simulink subsystem "TOAD_StateEstimator_2"  (R2026a)
settings: Solver=VariableStepAuto
undefined symbols (not defined in the file): constants6DoF, dt_SIM
settings Model: Creator=pplat  LastModifiedBy=alex2

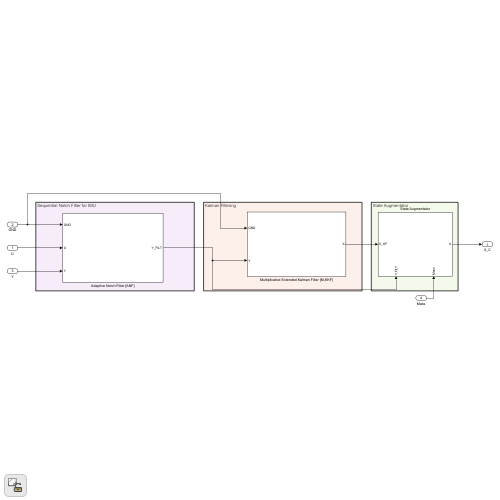
[thumbnail: Simulink's stored preview of the top-level diagram]
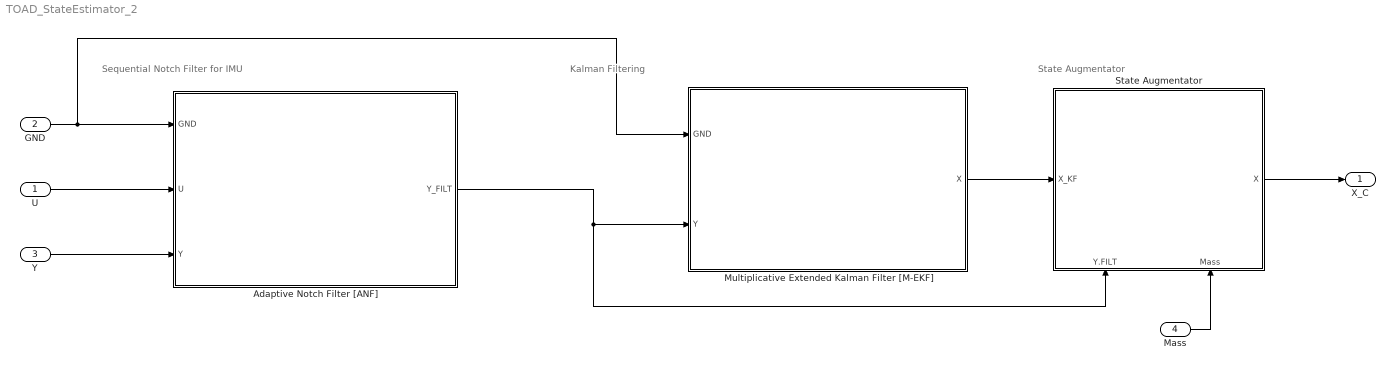
== system TOAD_StateEstimator_2 ==
  note: Kalman Filtering
  note: State Augmentator
  note: Sequential Notch Filter for IMU
  U : Inport  PortDimensions=[4, 1]
  GND : Inport  Port=2
  Y : Inport  Port=3  PortDimensions=[15, 1]
  Mass : Inport  Port=4
  Adaptive Notch Filter [ANF] : Subsystem
  Multiplicative Extended Kalman Filter [M-EKF] : Subsystem
  State Augmentator : Subsystem
      settings: PortSchema="{\"entries\":[{\"content\":{\"sides\":[{\"content\":{\"connectorIds\":[\"In1\"]},\"type\":\"ConnectorPlacement.EquallySpacedRectSide\",\"uuid\":\"bb6458aa-622a-4d42-b468-f616d6e302fe\"},{\"content\":{\"connectorIds\":[\"Out1\"],\"side\":\"RIGHT\"},\"type\":\"ConnectorPlacement.EquallySpacedRectSide\",\"uuid\":\"af8bade2-eb0a-4714-9db5-d33244eb3558\"},{\"content\":{\"side\":\"TOP\"},\"type\":\"ConnectorPlacement.EquallySpacedRectSide\",\"uuid\":\"05a7f106-e447-475e-b3b5-727cb0579a7b\"},{\"content\":{\"connectorIds\":[\"In2\",\"In3\"],\"side\":\"BOTTOM\"},\"type\":\"ConnectorPlacement.EquallySpacedRectSide\",\"uuid\":\"a6d44455-a42d-44f7-b37b-0d3db398c8f2\"}]},\"type\":\"ConnectorPlacement.EquallySpacedConnector\",\"uuid\":\"c6f62579-6b17-43b5-92f1-6190f0d9fd8b\"}],\"packageUris\":[\"http://schema.mathworks.com/mf0/Connector/R2020b\"],\"version\":\"1.0\"}"
  X_C : Outport
  wires:
  Adaptive Notch Filter [ANF]/1(Y_FILT) -> Multiplicative Extended Kalman Filter [M-EKF]/2(Y), State Augmentator/2(Y.FILT)
  Y/1 -> Adaptive Notch Filter [ANF]/3(Y)
  Multiplicative Extended Kalman Filter [M-EKF]/1(X) -> State Augmentator/1(X_KF)
  State Augmentator/1(X) -> X_C/1
  U/1 -> Adaptive Notch Filter [ANF]/2(U)
  GND/1 -> Multiplicative Extended Kalman Filter [M-EKF]/1(GND), Adaptive Notch Filter [ANF]/1(GND)
  Mass/1 -> State Augmentator/3(Mass)

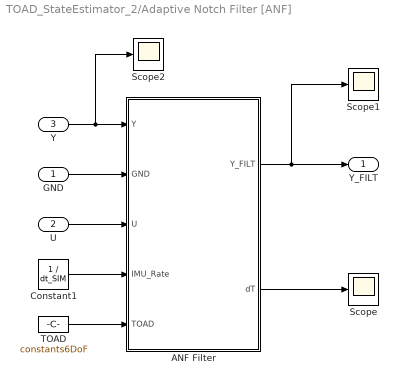
== system TOAD_StateEstimator_2/Adaptive Notch Filter [ANF] ==
  GND : Inport
  U : Inport  Port=2
  Y : Inport  Port=3
  ANF Filter : MATLAB Function  TreatAsAtomicUnit=on
  Constant1 : Constant  Value=1 / dt_SIM
  Scope : Scope
      settings: ActiveDisplayYMinimum=0.00014823443072048078  ActiveDisplayYMaximum=0.0020512828730928742  DataLoggingVariableName=ScopeData12
  Scope1 : Scope
      settings: ActiveDisplayYMinimum=-0.5661858721930958  ActiveDisplayYMaximum=0.35291049526280732  DataLoggingVariableName=ScopeData15
  Scope2 : Scope
      settings: ActiveDisplayYMinimum=-0.41652600912689441  ActiveDisplayYMaximum=0.41641236525722142  DataLoggingVariableName=ScopeData16
  TOAD : Constant  Value=constants6DoF  OutDataTypeStr=Bus: Vehicle_Bus
  Y_FILT : Outport
  wires:
  TOAD/1 -> ANF Filter/5(TOAD)
  ANF Filter/2(dT) -> Scope/1
  Constant1/1 -> ANF Filter/4(IMU_Rate)
  Y/1 -> ANF Filter/1(Y), Scope2/1
  U/1 -> ANF Filter/3(U)
  GND/1 -> ANF Filter/2(GND)
  ANF Filter/1(Y_FILT) -> Y_FILT/1, Scope1/1

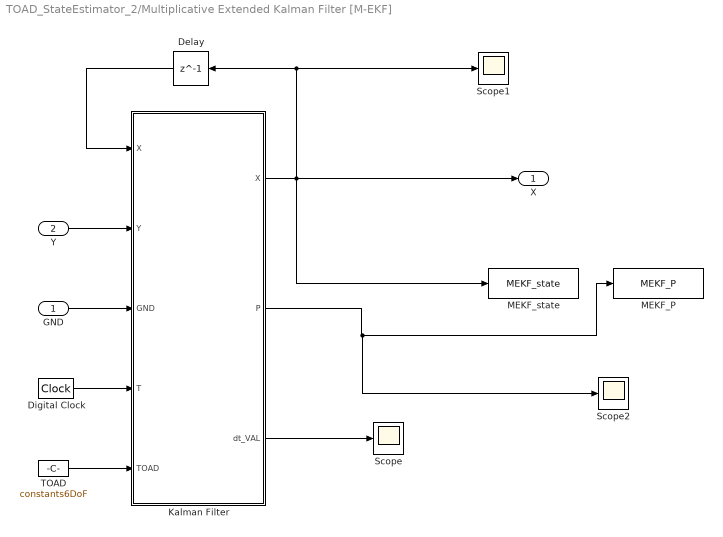
== system TOAD_StateEstimator_2/Multiplicative Extended Kalman Filter [M-EKF] ==
  GND : Inport
  Y : Inport  Port=2
  Delay : Delay  DelayLength=1  InitialCondition=[1; zeros(18,1)]
  Digital Clock : DigitalClock  SampleTime=dt_SIM
  Kalman Filter : MATLAB Function  TreatAsAtomicUnit=on
  MEKF_P : ToWorkspace  VariableName=MEKF_P  SaveFormat=Timeseries  SampleTime=-1
  MEKF_state : ToWorkspace  VariableName=MEKF_state  SaveFormat=Timeseries  SampleTime=-1
  Scope : Scope
      settings: ActiveDisplayYMinimum=-1  ActiveDisplayYMaximum=1
  Scope1 : Scope
      settings: ActiveDisplayYMinimum=-0.012655321840747358  ActiveDisplayYMaximum=0.022187884055420493  DataLoggingVariableName=ScopeData11
  Scope2 : Scope
      settings: ActiveDisplayYMinimum=-0.00099337090493864869  ActiveDisplayYMaximum=0.010796249758337241
  TOAD : Constant  Value=constants6DoF  OutDataTypeStr=Bus: Vehicle_Bus
  X : Outport
  wires:
  Kalman Filter/2(P) -> MEKF_P/1, Scope2/1
  GND/1 -> Kalman Filter/3(GND)
  TOAD/1 -> Kalman Filter/5(TOAD)
  Delay/1 -> Kalman Filter/1("X ")
  Y/1 -> Kalman Filter/2(Y)
  Kalman Filter/1(X) -> MEKF_state/1, X/1, Delay/1, Scope1/1
  Digital Clock/1 -> Kalman Filter/4(T)
  Kalman Filter/3(dt_VAL) -> Scope/1

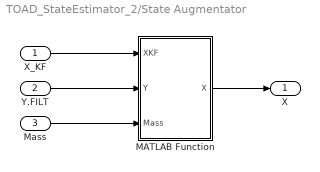
== system TOAD_StateEstimator_2/State Augmentator ==
  X_KF : Inport
  Y.FILT : Inport  Port=2
  Mass : Inport  Port=3
  MATLAB Function : MATLAB Function  TreatAsAtomicUnit=on
  X : Outport
  wires:
  Mass/1 -> MATLAB Function/3(Mass)
  Y.FILT/1 -> MATLAB Function/2(Y)
  MATLAB Function/1(X) -> X/1
  X_KF/1 -> MATLAB Function/1(XKF)

== matlab function TOAD_StateEstimator_2/Multiplicative Extended Kalman Filter [M-EKF]/Kalman Filter ==
  data: X input; Y input; GND input; X output; T input; TOAD input; P output; dt_VAL output
function [X, P, dt_VAL] = MEKF(X, Y, GND, T, TOAD)

    % Measure simulation timestep
    persistent dt lastT lastP
    if isempty(dt)
        dt = 0;
        lastT = 0;
        lastP = eye(18);
    end
    dt = T - lastT;
    lastT = T;
    
    if GND
        [X, lastP] = GroundEstimator(X, TOAD, Y, dt);
    else
        %% FlightEstimator.m
        % [X, lastP(1:9, 1:9)] = FlightEstimator(X, TOAD, Y, dt, lastP(1:9, 1:9));
        % Liftoff = 1;

        %% FlightEstimator2.m
        [X, lastP(1:12, 1:12)] = FlightEstimator2(X, TOAD, Y, dt, lastP(1:12, 1:12));
    end
    P = diag(lastP);
    dt_VAL = dt;
end
    %X = EstimateStateFCN(X, ASTRAv2, Y, dt, GND);

== matlab function TOAD_StateEstimator_2/State Augmentator/MATLAB Function ==
  data: XKF input; X output; Y input; Mass input
function X = StateAUG(XKF, Y, Mass)

% Change Filter State to Controls State
% ADD MASS ESTIMATION
X = [XKF(1:4); XKF(5:7); XKF(8:10); Y(4:6) - XKF(11:13); Mass(1:2)];

== matlab function TOAD_StateEstimator_2/Adaptive Notch Filter [ANF]/ANF Filter ==
  data: Y input; Y_FILT output; GND input; U input; IMU_Rate input; dT output; TOAD input
function [Y_FILT, dT] = ANF_Filter(Y, GND, U, IMU_Rate, TOAD)

% Extract IMU
IMU = Y(1:9);
dT = 1 / IMU_Rate;

% Thrust PCT
THRUST = U(3) / TOAD.MaxThrust * 100;

% ANF Filter
ANF_IMU = DigitalNF(IMU, 0, THRUST, dT);

% Combine (FILTER CURRENTLY OFF)
Y_FILT = [ANF_IMU; Y(10:15)];
